simulink model "Channelizer_demo"  (R2023b)
settings: Solver=VariableStepAuto  StartTime=0.0  StopTime=inf  RelTol=1e-3
PostLoadFcn:
  | TT = numerictype(1,16,15);
  | FF = fimath('RoundingMethod','Nearest','OverflowAction','Saturate');
  | mdl = channelizer_init(TT, FF);
  | channelizer = channelizer_model(mdl, TT, FF );
  | Ts = 16*(7/4)/8.75e9;
  | ch_filt_coef = rcosdesign(0.22,4,28,'normal');
  | ch_filt_coef = 28 * ch_filt_coef / sum(ch_filt_coef(:));
  | channelizer_demo_init;
values from neighbouring files (symbols this model uses):
  ch0_en = 0    [channelizer_demo_init.m]    (also in init.m)
  ch0_qam = 0    [channelizer_demo_init.m]    (also in init.m)
  ch0_swp = 0    [channelizer_demo_init.m]    (also in init.m)
  ch10_en = 0    [channelizer_demo_init.m]    (also in init.m)
  ch10_qam = 0    [channelizer_demo_init.m]    (also in init.m)
  ch10_swp = 0    [channelizer_demo_init.m]    (also in init.m)
  ch11_en = 0    [channelizer_demo_init.m]    (also in init.m)
  ch11_qam = 0    [channelizer_demo_init.m]    (also in init.m)
  ch11_swp = 0    [channelizer_demo_init.m]    (also in init.m)
  ch12_en = 0    [channelizer_demo_init.m]    (also in init.m)
  ch12_qam = 0    [channelizer_demo_init.m]    (also in init.m)
  ch12_swp = 0    [channelizer_demo_init.m]    (also in init.m)
  ch13_en = 0    [channelizer_demo_init.m]    (also in init.m)
  ch13_qam = 0    [channelizer_demo_init.m]    (also in init.m)
  ch13_swp = 0    [channelizer_demo_init.m]    (also in init.m)
  ch14_en = 0    [channelizer_demo_init.m]    (also in init.m)
  ch14_qam = 0    [channelizer_demo_init.m]    (also in init.m)
  ch14_swp = 0    [channelizer_demo_init.m]    (also in init.m)
  ch15_en = 0    [channelizer_demo_init.m]    (also in init.m)
  ch15_qam = 0    [channelizer_demo_init.m]    (also in init.m)
  ch15_swp = 0    [channelizer_demo_init.m]    (also in init.m)
  ch1_en = 1    [channelizer_demo_init.m]    (also in init.m)
  ch1_qam = 0    [channelizer_demo_init.m]    (also in init.m)
  ch1_swp = 0    [channelizer_demo_init.m]    (also in init.m)
  ch2_en = 1    [channelizer_demo_init.m]    (also in init.m)
  ch2_qam = 0    [channelizer_demo_init.m]    (also in init.m)
  ch2_swp = 0    [channelizer_demo_init.m]    (also in init.m)
  ch3_en = 0    [channelizer_demo_init.m]    (also in init.m)
  ch3_qam = 0    [channelizer_demo_init.m]    (also in init.m)
  ch3_swp = 0    [channelizer_demo_init.m]    (also in init.m)
  ch4_en = 0    [channelizer_demo_init.m]    (also in init.m)
  ch4_qam = 0    [channelizer_demo_init.m]    (also in init.m)
  ch4_swp = 0    [channelizer_demo_init.m]    (also in init.m)
  ch5_en = 1    [channelizer_demo_init.m]    (also in init.m)
  ch5_qam = 1    [channelizer_demo_init.m]    (also in init.m)
  ch5_swp = 0    [channelizer_demo_init.m]    (also in init.m)
  ch6_en = 1    [channelizer_demo_init.m]    (also in init.m)
  ch6_qam = 1    [channelizer_demo_init.m]    (also in init.m)
  ch6_swp = 0    [channelizer_demo_init.m]    (also in init.m)
  ch7_en = 0    [channelizer_demo_init.m]    (also in init.m)
  ch7_qam = 0    [channelizer_demo_init.m]    (also in init.m)
  ch7_swp = 0    [channelizer_demo_init.m]    (also in init.m)
  ch8_en = 0    [channelizer_demo_init.m]    (also in init.m)
  ch8_qam = 0    [channelizer_demo_init.m]    (also in init.m)
  ch8_swp = 0    [channelizer_demo_init.m]    (also in init.m)
  ch9_en = 0    [channelizer_demo_init.m]    (also in init.m)
  ch9_qam = 0    [channelizer_demo_init.m]    (also in init.m)
  ch9_swp = 0    [channelizer_demo_init.m]    (also in init.m)
  spec1_ch = 1    [channelizer_demo_init.m]    (also in init.m)
  spec2_ch = 2    [channelizer_demo_init.m]    (also in init.m)
  spec3_ch = 5    [channelizer_demo_init.m]    (also in init.m)
  spec4_ch = 6    [channelizer_demo_init.m]    (also in init.m)
  swp_rate0 = 0    [channelizer_demo_init.m]    (also in init.m)
  swp_rate1 = 0    [channelizer_demo_init.m]    (also in init.m)
  swp_rate10 = 0    [channelizer_demo_init.m]    (also in init.m)
  swp_rate11 = 0    [channelizer_demo_init.m]    (also in init.m)
  swp_rate12 = 0    [channelizer_demo_init.m]    (also in init.m)
  swp_rate13 = 0    [channelizer_demo_init.m]    (also in init.m)
  swp_rate14 = 0    [channelizer_demo_init.m]    (also in init.m)
  swp_rate15 = 0    [channelizer_demo_init.m]    (also in init.m)
  swp_rate2 = 0    [channelizer_demo_init.m]    (also in init.m)
  swp_rate3 = 0    [channelizer_demo_init.m]    (also in init.m)
  swp_rate4 = 0    [channelizer_demo_init.m]    (also in init.m)
  swp_rate5 = 0    [channelizer_demo_init.m]    (also in init.m)
  swp_rate6 = 0    [channelizer_demo_init.m]    (also in init.m)
  swp_rate7 = 0    [channelizer_demo_init.m]    (also in init.m)
  swp_rate8 = 0    [channelizer_demo_init.m]    (also in init.m)
  swp_rate9 = 0    [channelizer_demo_init.m]    (also in init.m)
undefined symbols (not defined in the file or in its folder): S, vsva2197, xcvc1902
libraries: aieUtilities x39, aieBasic x34, dspswit3 x16, dspsigops x16, hlsBasic x3, vmcUtilities x1, commchan3 x1
(part 1 of 3)
settings Model: Creator=robg  LastModifiedBy=rbuz
settings DataIOCC: SaveFormat=Array  SaveOutput=off  SignalLogging=off  DSMLogging=off  SaveTime=off
settings OptimizationCC: ReuseModelBlockBuffer=off
settings DebuggingCC: ParameterOverflowMsg=none  ParameterPrecisionLossMsg=none  UnconnectedInputMsg=warning  UnconnectedOutputMsg=warning  UnconnectedLineMsg=warning
settings ModelReferenceCC: EnableRefExpFcnMdlSchedulingChecks=on
settings RTWCC: DLArmComputeVersion=19.05

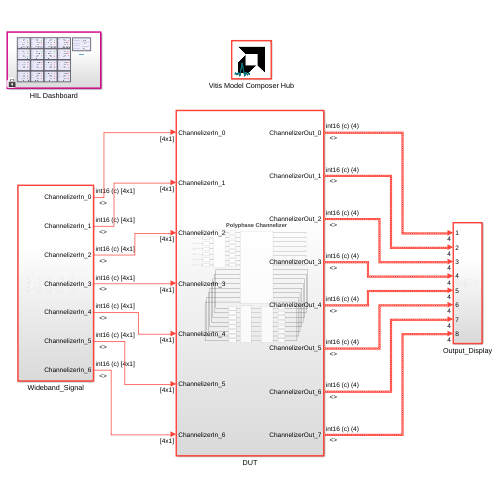
[thumbnail: Simulink's stored preview of the top-level diagram]
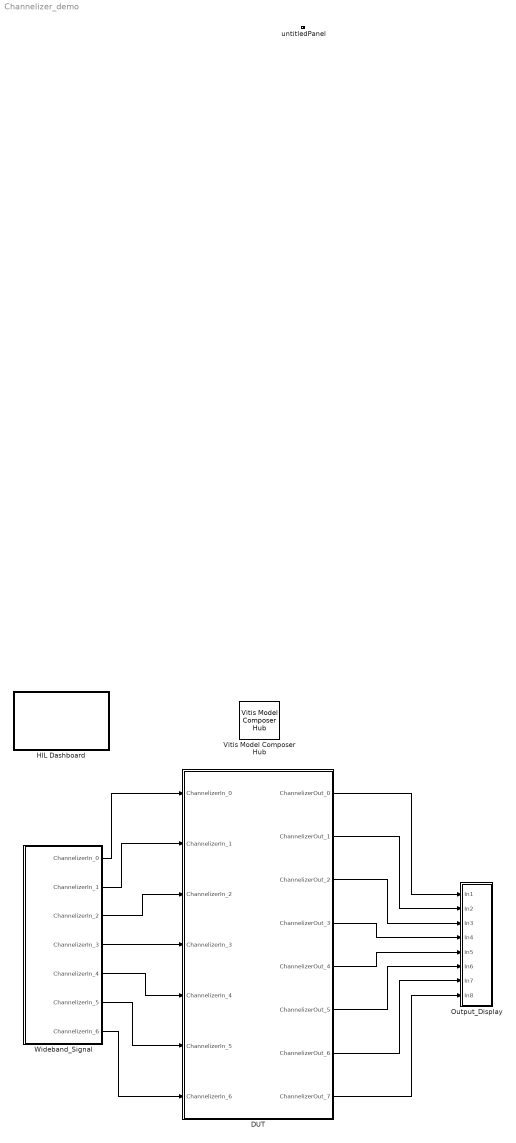
== system Channelizer_demo ==
  DUT : Subsystem
  HIL Dashboard : Subsystem
  Output_Display : Subsystem
  Vitis Model Composer Hub : vmcUtilities/Vitis Model Composer Hub  Tag=genX  CodeGeneration=off  SubsystemName=Channelizer  TargetDirectory=./code  exportDesign=off  analyzeDesign=off  validateDesignOnHw=off  ExportType=HW Code  IpVendor=xilinx.com  IpLibrary=hls  IpVersion=1.0  IpHWLanguage=Verilog  AieCompilerOptions={}  AieSimulatorOptions={}  CreateTestbench=off  TestbenchStackSize=10  RunRtlSim=off  RunCSim=off  RunAieSim=off  AieSimTimeout=50000  RunAieSimProfiling=off  LaunchVitisAnalyzer=off  PlotOutput=off  RunX86Sim=off  X86SimTimeout=10  GenHwImage=off  GenLibadfXo=off  GenHwValidationCode=off  PlatformType=Specify Platform  Platform=/proj/xbuilds/SWIP/2023.2_0918_2207/installs/lin64/Vitis/2023.2/base_platforms/xilinx_vck190_base_202320_1/xilinx_vck190_base_202320_1.xpfm  HwSystemType=Baremetal  HwValidationTarget=hw_emu  ProjDevice=Versal VCK190 Evaluation Platform (xcvc1902-vsva2197-2MP-e-S)  ProjDevicePart=xcvc1902-vsva2197-2MP-e-S  AIEType=AIE  SamplePeriod=-1  ClockFrequency=200  DataPathParallelism=1  xilinxfamily=versalaicore  part=xcvc1902  speed=-2MP-e-S  package=vsva2197  directory=./netlist  testbench=off  incr_netlist=off  synthesis_tool=Vivado  clock_wrapper=Clock Enables  dbl_ovrd=According to Block Masks  dcm_input_clock_period=10  sysclk_period=10  simulink_period=1  eval_field=0  LogFileName=/proj/xcoswmktg/robg/git/vmc_examples/gitent/Examples/AIENGINE_plus_PL/AIE_HLS/Channelizer/code/model_composer.log  NThreads=4
  Wideband_Signal : Subsystem
  untitledPanel : Subsystem  Tag=HiddenForWebPanel  IsWebBlockPanel=on
  wires:
  Wideband_Signal/7(ChannelizerIn_6) -> DUT/7(ChannelizerIn_6)
  Wideband_Signal/6(ChannelizerIn_5) -> DUT/6(ChannelizerIn_5)
  Wideband_Signal/5(ChannelizerIn_4) -> DUT/5(ChannelizerIn_4)
  Wideband_Signal/4(ChannelizerIn_3) -> DUT/4(ChannelizerIn_3)
  Wideband_Signal/3(ChannelizerIn_2) -> DUT/3(ChannelizerIn_2)
  Wideband_Signal/2(ChannelizerIn_1) -> DUT/2(ChannelizerIn_1)
  Wideband_Signal/1(ChannelizerIn_0) -> DUT/1(ChannelizerIn_0)
  DUT/1(ChannelizerOut_0) -> Output_Display/1(In1)
  DUT/2(ChannelizerOut_1) -> Output_Display/2(In2)
  DUT/3(ChannelizerOut_2) -> Output_Display/3(In3)
  DUT/4(ChannelizerOut_3) -> Output_Display/4(In4)
  DUT/5(ChannelizerOut_4) -> Output_Display/5(In5)
  DUT/6(ChannelizerOut_5) -> Output_Display/6(In6)
  DUT/7(ChannelizerOut_6) -> Output_Display/7(In7)
  DUT/8(ChannelizerOut_7) -> Output_Display/8(In8)

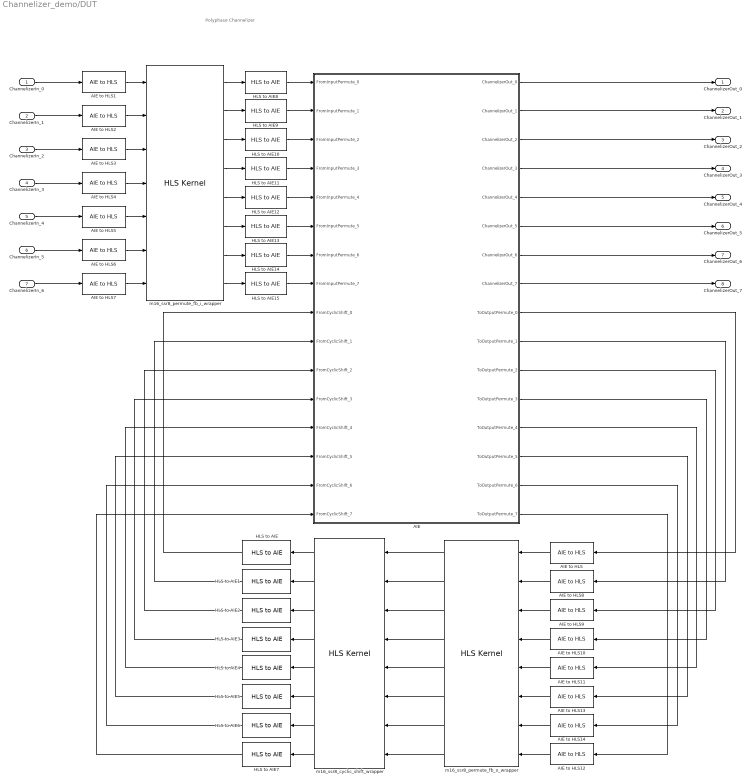
== system Channelizer_demo/DUT ==
  note: Polyphase Channelizer
  ChannelizerIn_0 : Inport
  ChannelizerIn_1 : Inport  Port=2
  ChannelizerIn_2 : Inport  Port=3
  ChannelizerIn_3 : Inport  Port=4
  ChannelizerIn_4 : Inport  Port=5
  ChannelizerIn_5 : Inport  Port=6
  ChannelizerIn_6 : Inport  Port=7
  AIE : Subsystem
  AIE to HLS{,1..14} (15 alike) : aieUtilities/AIE to HLS  OutputType=ufix128  OutputSize=1
  HLS to AIE{,1..15} (16 alike) : aieUtilities/HLS to AIE  OutputType=cint16  OutputSize=4
  m16_ssr8_cyclic_shift_wrapper : hlsBasic/HLS Kernel  PortNames={'return'; 'sig0_i'; 'sig1_i'; 'sig2_i'; 'sig3_i'; 'sig4_i'; 'sig5_i'; 'sig6_i'; 'sig7_i'; 'sig0_o'; 'sig1_o'; 'sig2_o'; 'sig3_o'; 'sig4_o'; 'sig5_o'; 'sig6_o'; 'sig7_o'}  PortSerializedTypes={'{Bv}'; '{R{Thls::stream{2{t{Tap_uint{1{t{}128}}}}{t{}0}}}}'; '{R{Thls::stream{2{t{Tap_uint{1{t{}128}}}}{t{}0}}}}'; '{R{Thls::stream{2{t{Tap_uint{1{t{}128}}}}{t{}0}}}}'; '{R{Thls::stream{2{t{Tap_uint{1{t{}128}}}}{t{}0}}}}'; '{R{Thls::stream{2{t{Tap_uint{1{t{}128}}}}{t{}0}}}}'; '{R{Thls::stream{2{t{Tap_uint{1{t{}128}}}}{t{}0}}}}'; '{R{Thls::stream{2{t{Tap_uint{1{t{}128}}}}{t{}0}}}}'; '{R{Thls::stream{2{t{Tap_uint{1{t{}128}}}}{t{}0}}}}'; '{R{Thls::stream{2{t{Tap_uint{1{t{}128}}}}{t{}0}}}}'; '{R{Thls::stream{2{t{Tap_uint{1{t{}128}}}}{t{}0}}}}'; '{R{Thls::stream{2{t{Tap_uint{1{t{}128}}}}{t{}0}}}}'; '{R{Thls::stream{2{t{Tap_uint{1{t{}128}}}}{t{}0}}}}'; '{R{Thls::stream{2{t{Tap_uint{1{t{}128}}}}{t{}0}}}}'; '{R{Thls::stream{2{t{Tap_uint{1{t{}128}}}}{t{}0}}}}'; '{R{Thls::stream{2{t{Tap_uint{1{t{}128}}}}{t{}0}}}}'; '{R{Thls::stream{2{t{Tap_uint{1{t{}128}}}}{t{}0}}}}'}  FunctionTemplateSpecKind=none  FunctionTemplateParamNames={}  FunctionTemplateParamKinds={}  FunctionTemplateParamTypes={}  FunctionTemplateParamValues={}  PortSynchronicities={'auto'; 'auto'; 'auto'; 'auto'; 'auto'; 'auto'; 'auto'; 'auto'; 'auto'; 'auto'; 'auto'; 'auto'; 'auto'; 'auto'; 'auto'; 'auto'}  PortSignalSizes={0.000000000000000000e+00; 0.000000000000000000e+00; 0.000000000000000000e+00; 0.000000000000000000e+00; 0.000000000000000000e+00; 0.000000000000000000e+00; 0.000000000000000000e+00; 0.000000000000000000e+00; 1.000000000000000000e+00; 1.000000000000000000e+00; 1.000000000000000000e+00; 1.000000000000000000e+00; 1.000000000000000000e+00; 1.000000000000000000e+00; 1.000000000000000000e+00; 1.000000000000000000e+00}  PortParameterValues={}  FunctionTemplateParams={}  FunctionTemplateParamsEnables={}  FunctionTemplateParamsVisible=off  FunctionDeclTypeOptions=C[1 1]@t7@<empty>  PortAttributesTable={ 'Input', 'sig0_i', 'hls::stream< ap_uint< 128 >, 0 > &', '', ''; 'Input', 'sig1_i', 'hls::stream< ap_uint< 128 >, 0 > &', '', ''; 'Input', 'sig2_i', 'hls::stream< ap_uint< 128 >, 0 > &', '', ''; 'Input', 'sig3_i', 'hls::stream< ap_uint< 128 >, 0 > &', '', ''; 'Input', 'sig4_i', 'hls::stream< ap_uint< 128 >, 0 > &', '', ''; 'Input', 'sig5_i', 'hls::stream< ap_uint< 128 >, 0 > &', '', ''; 'Input', 'sig6_i', 'hls::stream< ap_uint< 128 >, 0 > &', '', ''; 'Input', 'sig7_i', 'hls::stream< ap_uint< 128 >, 0 > &', '', ''; 'Output', 'sig0_o', 'hls::stream< ap_uint< 128 >, 0 > &', '', '1'; 'Output', 'sig1_o', 'hls::stream< ap_uint< 128 >, 0 > &', '', '1'; 'Output', 'sig2_o', 'hls::stream< ap_uint< 128 >, 0 > &', '', '1'; 'Output', 'sig3_o', 'hls::stream< ap_uint< 128 >, 0 > &', '', '1'; 'Output', 'sig4_o', 'hls::stream< ap_uint< 128 >, 0 > &', '', '1'; 'Output', 'sig5_o', 'hls::stream< ap_uint< 128 >, 0 > &', '', '1'; 'Output', 'sig6_o', 'hls::stream< ap_uint< 128 >, 0 > &', '', '1'; 'Output', 'sig7_o', 'hls::stream< ap_uint< 128 >, 0 > &', '', '1' }  PortAttributesEnablement={'off', 'off', 'off', 'off', 'off';'off', 'off', 'off', 'off', 'off';'off', 'off', 'off', 'off', 'off';'off', 'off', 'off', 'off', 'off';'off', 'off', 'off', 'off', 'off';'off', 'off', 'off', 'off', 'off';'off', 'off', 'off', 'off', 'off';'off', 'off', 'off', 'off', 'off';'off', 'off', 'off', 'off', 'on';'off', 'off', 'off', 'off', 'on';'off', 'off', 'off', 'off', 'on';'off', 'off', 'off', 'off', 'on';'off', 'off', 'off', 'off', 'on';'off', 'off', 'off', 'off', 'on';'off', 'off', 'off', 'off', 'on';'off', 'off', 'off', 'off', 'on'}  PortParametersTable={}  SampleTime=-1  PortDirectionTable={ 'sig0_i', 'hls::stream< ap_uint< 128 >, 0 > &', 'Input', 'Port'; 'sig1_i', 'hls::stream< ap_uint< 128 >, 0 > &', 'Input', 'Port'; 'sig2_i', 'hls::stream< ap_uint< 128 >, 0 > &', 'Input', 'Port'; 'sig3_i', 'hls::stream< ap_uint< 128 >, 0 > &', 'Input', 'Port'; 'sig4_i', 'hls::stream< ap_uint< 128 >, 0 > &', 'Input', 'Port'; 'sig5_i', 'hls::stream< ap_uint< 128 >, 0 > &', 'Input', 'Port'; 'sig6_i', 'hls::stream< ap_uint< 128 >, 0 > &', 'Input', 'Port'; 'sig7_i', 'hls::stream< ap_uint< 128 >, 0 > &', 'Input', 'Port'; 'sig0_o', 'hls::stream< ap_uint< 128 >, 0 > &', 'Output', 'Port'; 'sig1_o', 'hls::stream< ap_uint< 128 >, 0 > &', 'Output', 'Port'; 'sig2_o', 'hls::stream< ap_uint< 128 >, 0 > &', 'Output', 'Port'; 'sig3_o', 'hls::stream< ap_uint< 128 >, 0 > &', 'Output', 'Port'; 'sig4_o', 'hls::stream< ap_uint< 128 >, 0 > &', 'Output', 'Port'; 'sig5_o', 'hls::stream< ap_uint< 128 >, 0 > &', 'Output', 'Port'; 'sig6_o', 'hls::stream< ap_uint< 128 >, 0 > &', 'Output', 'Port'; 'sig7_o', 'hls::stream< ap_uint< 128 >, 0 > &', 'Output', 'Port' }  PortDirectionTabVisible=on  ArgDirections={1.000000000000000000e+00; 1.000000000000000000e+00; 1.000000000000000000e+00; 1.000000000000000000e+00; 1.000000000000000000e+00; 1.000000000000000000e+00; 1.000000000000000000e+00; 1.000000000000000000e+00; 2.000000000000000000e+00; 2.000000000000000000e+00; 2.000000000000000000e+00; 2.000000000000000000e+00; 2.000000000000000000e+00; 2.000000000000000000e+00; 2.000000000000000000e+00; 2.000000000000000000e+00}  ArgInterfaceTypes={1.000000000000000000e+00; 1.000000000000000000e+00; 1.000000000000000000e+00; 1.000000000000000000e+00; 1.000000000000000000e+00; 1.000000000000000000e+00; 1.000000000000000000e+00; 1.000000000000000000e+00; 1.000000000000000000e+00; 1.000000000000000000e+00; 1.000000000000000000e+00; 1.000000000000000000e+00; 1.000000000000000000e+00; 1.000000000000000000e+00; 1.000000000000000000e+00; 1.000000000000000000e+00}  FunctionIndex=1  FormalArgDecls={'hls::stream< ap_uint< 128 >, 0 > & sig0_i', 'hls::stream< ap_uint< 128 >, 0 > & sig1_i', 'hls::stream< ap_uint< 128 >, 0 > & sig2_i', 'hls::stream< ap_uint< 128 >, 0 > & sig3_i', 'hls::stream< ap_uint< 128 >, 0 > & sig4_i', 'hls::stream< ap_uint< 128 >, 0 > & sig5_i', 'hls::stream< ap_uint< 128 >, 0 > & sig6_i', 'hls::stream< ap_uint< 128 >, 0 > & sig7_i', 'hls::stream< ap_uint< 128 >, 0 > & sig0_o', 'hls::stream< ap_uint< 128 >, 0 > & sig1_o', 'hls::stream< ap_uint< 128 >, 0 > & sig2_o', 'hls::stream< ap_uint< 128 >, 0 > & sig3_o', 'hls::stream< ap_uint< 128 >, 0 > & sig4_o', 'hls::stream< ap_uint< 128 >, 0 > & sig5_o', 'hls::stream< ap_uint< 128 >, 0 > & sig6_o', 'hls::stream< ap_uint< 128 >, 0 > & sig7_o'}  SimLibPath=''  FunctionTabVisible=on  FunctionDescription=void m16_ssr8_cyclic_shift_wrapper(hls::stream< ap_uint< 128 >, 0 > & sig0_i, hls::stream< ap_uint< 128 >, 0 > & sig1_i, hls::stream< ap_uint< 128 >, 0 > & sig2_i, hls::stream< ap_uint< 128 >, 0 > & sig3_i, hls::stream< ap_uint< 128 >, 0 > & sig4_i, hls::stream< ap_uint< 128 >, 0 > & sig5_i, hls::stream< ap_uint< 128 >, 0 > & sig6_i, hls::stream< ap_uint< 128 >, 0 > & sig7_i, hls::stream< ap_uint< 128 >, 0 > & sig0_o, hls::stream< ap_uint< 128 >, 0 > & sig1_o, hls::stream< ap_uint< 128 >, 0 > & sig2_o, hls::stream< ap_uint< 128 >, 0 > & sig3_o, hls::stream< ap_uint< 128 >, 0 > & sig4_o, hls::stream< ap_uint< 128 >, 0 > & sig5_o, hls::stream< ap_uint< 128 >, 0 > & sig6_o, hls::stream< ap_uint< 128 >, 0 > & sig7_o)  blockJsonConstraints=[]  deprecateConstraints=0  KernelHeaderFile=hls/m16_ssr8_cyclic_shift.h  KernelFunction=m16_ssr8_cyclic_shift_wrapper  KernelFunctionSelect=<empty>  KernelSourceFile=hls/m16_ssr8_cyclic_shift.cpp  KernelSearchPaths={}  PreProcOptions={}
  m16_ssr8_permute_fb_i_wrapper : hlsBasic/HLS Kernel  PortNames={'return'; 'sig0_i'; 'sig1_i'; 'sig2_i'; 'sig3_i'; 'sig4_i'; 'sig5_i'; 'sig6_i'; 'sig0_o'; 'sig1_o'; 'sig2_o'; 'sig3_o'; 'sig4_o'; 'sig5_o'; 'sig6_o'; 'sig7_o'}  PortSerializedTypes={'{Bv}'; '{R{Thls::stream{2{t{Tap_uint{1{t{}128}}}}{t{}0}}}}'; '{R{Thls::stream{2{t{Tap_uint{1{t{}128}}}}{t{}0}}}}'; '{R{Thls::stream{2{t{Tap_uint{1{t{}128}}}}{t{}0}}}}'; '{R{Thls::stream{2{t{Tap_uint{1{t{}128}}}}{t{}0}}}}'; '{R{Thls::stream{2{t{Tap_uint{1{t{}128}}}}{t{}0}}}}'; '{R{Thls::stream{2{t{Tap_uint{1{t{}128}}}}{t{}0}}}}'; '{R{Thls::stream{2{t{Tap_uint{1{t{}128}}}}{t{}0}}}}'; '{R{Thls::stream{2{t{Tap_uint{1{t{}128}}}}{t{}0}}}}'; '{R{Thls::stream{2{t{Tap_uint{1{t{}128}}}}{t{}0}}}}'; '{R{Thls::stream{2{t{Tap_uint{1{t{}128}}}}{t{}0}}}}'; '{R{Thls::stream{2{t{Tap_uint{1{t{}128}}}}{t{}0}}}}'; '{R{Thls::stream{2{t{Tap_uint{1{t{}128}}}}{t{}0}}}}'; '{R{Thls::stream{2{t{Tap_uint{1{t{}128}}}}{t{}0}}}}'; '{R{Thls::stream{2{t{Tap_uint{1{t{}128}}}}{t{}0}}}}'; '{R{Thls::stream{2{t{Tap_uint{1{t{}128}}}}{t{}0}}}}'}  FunctionTemplateSpecKind=none  FunctionTemplateParamNames={}  FunctionTemplateParamKinds={}  FunctionTemplateParamTypes={}  FunctionTemplateParamValues={}  PortSynchronicities={'auto'; 'auto'; 'auto'; 'auto'; 'auto'; 'auto'; 'auto'; 'auto'; 'auto'; 'auto'; 'auto'; 'auto'; 'auto'; 'auto'; 'auto'}  PortSignalSizes={0.000000000000000000e+00; 0.000000000000000000e+00; 0.000000000000000000e+00; 0.000000000000000000e+00; 0.000000000000000000e+00; 0.000000000000000000e+00; 0.000000000000000000e+00; 1.000000000000000000e+00; 1.000000000000000000e+00; 1.000000000000000000e+00; 1.000000000000000000e+00; 1.000000000000000000e+00; 1.000000000000000000e+00; 1.000000000000000000e+00; 1.000000000000000000e+00}  PortParameterValues={}  FunctionTemplateParams={}  FunctionTemplateParamsEnables={}  FunctionTemplateParamsVisible=off  FunctionDeclTypeOptions=C[1 1]@t7@<empty>  PortAttributesTable={ 'Input', 'sig0_i', 'hls::stream< ap_uint< 128 >, 0 > &', '', ''; 'Input', 'sig1_i', 'hls::stream< ap_uint< 128 >, 0 > &', '', ''; 'Input', 'sig2_i', 'hls::stream< ap_uint< 128 >, 0 > &', '', ''; 'Input', 'sig3_i', 'hls::stream< ap_uint< 128 >, 0 > &', '', ''; 'Input', 'sig4_i', 'hls::stream< ap_uint< 128 >, 0 > &', '', ''; 'Input', 'sig5_i', 'hls::stream< ap_uint< 128 >, 0 > &', '', ''; 'Input', 'sig6_i', 'hls::stream< ap_uint< 128 >, 0 > &', '', ''; 'Output', 'sig0_o', 'hls::stream< ap_uint< 128 >, 0 > &', '', '1'; 'Output', 'sig1_o', 'hls::stream< ap_uint< 128 >, 0 > &', '', '1'; 'Output', 'sig2_o', 'hls::stream< ap_uint< 128 >, 0 > &', '', '1'; 'Output', 'sig3_o', 'hls::stream< ap_uint< 128 >, 0 > &', '', '1'; 'Output', 'sig4_o', 'hls::stream< ap_uint< 128 >, 0 > &', '', '1'; 'Output', 'sig5_o', 'hls::stream< ap_uint< 128 >, 0 > &', '', '1'; 'Output', 'sig6_o', 'hls::stream< ap_uint< 128 >, 0 > &', '', '1'; 'Output', 'sig7_o', 'hls::stream< ap_uint< 128 >, 0 > &', '', '1' }  PortAttributesEnablement={'off', 'off', 'off', 'off', 'off';'off', 'off', 'off', 'off', 'off';'off', 'off', 'off', 'off', 'off';'off', 'off', 'off', 'off', 'off';'off', 'off', 'off', 'off', 'off';'off', 'off', 'off', 'off', 'off';'off', 'off', 'off', 'off', 'off';'off', 'off', 'off', 'off', 'on';'off', 'off', 'off', 'off', 'on';'off', 'off', 'off', 'off', 'on';'off', 'off', 'off', 'off', 'on';'off', 'off', 'off', 'off', 'on';'off', 'off', 'off', 'off', 'on';'off', 'off', 'off', 'off', 'on';'off', 'off', 'off', 'off', 'on'}  PortParametersTable={}  SampleTime=-1  PortDirectionTable={ 'sig0_i', 'hls::stream< ap_uint< 128 >, 0 > &', 'Input', 'Port'; 'sig1_i', 'hls::stream< ap_uint< 128 >, 0 > &', 'Input', 'Port'; 'sig2_i', 'hls::stream< ap_uint< 128 >, 0 > &', 'Input', 'Port'; 'sig3_i', 'hls::stream< ap_uint< 128 >, 0 > &', 'Input', 'Port'; 'sig4_i', 'hls::stream< ap_uint< 128 >, 0 > &', 'Input', 'Port'; 'sig5_i', 'hls::stream< ap_uint< 128 >, 0 > &', 'Input', 'Port'; 'sig6_i', 'hls::stream< ap_uint< 128 >, 0 > &', 'Input', 'Port'; 'sig0_o', 'hls::stream< ap_uint< 128 >, 0 > &', 'Output', 'Port'; 'sig1_o', 'hls::stream< ap_uint< 128 >, 0 > &', 'Output', 'Port'; 'sig2_o', 'hls::stream< ap_uint< 128 >, 0 > &', 'Output', 'Port'; 'sig3_o', 'hls::stream< ap_uint< 128 >, 0 > &', 'Output', 'Port'; 'sig4_o', 'hls::stream< ap_uint< 128 >, 0 > &', 'Output', 'Port'; 'sig5_o', 'hls::stream< ap_uint< 128 >, 0 > &', 'Output', 'Port'; 'sig6_o', 'hls::stream< ap_uint< 128 >, 0 > &', 'Output', 'Port'; 'sig7_o', 'hls::stream< ap_uint< 128 >, 0 > &', 'Output', 'Port' }  PortDirectionTabVisible=on  ArgDirections={1.000000000000000000e+00; 1.000000000000000000e+00; 1.000000000000000000e+00; 1.000000000000000000e+00; 1.000000000000000000e+00; 1.000000000000000000e+00; 1.000000000000000000e+00; 2.000000000000000000e+00; 2.000000000000000000e+00; 2.000000000000000000e+00; 2.000000000000000000e+00; 2.000000000000000000e+00; 2.000000000000000000e+00; 2.000000000000000000e+00; 2.000000000000000000e+00}  ArgInterfaceTypes={1.000000000000000000e+00; 1.000000000000000000e+00; 1.000000000000000000e+00; 1.000000000000000000e+00; 1.000000000000000000e+00; 1.000000000000000000e+00; 1.000000000000000000e+00; 1.000000000000000000e+00; 1.000000000000000000e+00; 1.000000000000000000e+00; 1.000000000000000000e+00; 1.000000000000000000e+00; 1.000000000000000000e+00; 1.000000000000000000e+00; 1.000000000000000000e+00}  FunctionIndex=1  FormalArgDecls={'hls::stream< ap_uint< 128 >, 0 > & sig0_i', 'hls::stream< ap_uint< 128 >, 0 > & sig1_i', 'hls::stream< ap_uint< 128 >, 0 > & sig2_i', 'hls::stream< ap_uint< 128 >, 0 > & sig3_i', 'hls::stream< ap_uint< 128 >, 0 > & sig4_i', 'hls::stream< ap_uint< 128 >, 0 > & sig5_i', 'hls::stream< ap_uint< 128 >, 0 > & sig6_i', 'hls::stream< ap_uint< 128 >, 0 > & sig0_o', 'hls::stream< ap_uint< 128 >, 0 > & sig1_o', 'hls::stream< ap_uint< 128 >, 0 > & sig2_o', 'hls::stream< ap_uint< 128 >, 0 > & sig3_o', 'hls::stream< ap_uint< 128 >, 0 > & sig4_o', 'hls::stream< ap_uint< 128 >, 0 > & sig5_o', 'hls::stream< ap_uint< 128 >, 0 > & sig6_o', 'hls::stream< ap_uint< 128 >, 0 > & sig7_o'}  SimLibPath=''  FunctionTabVisible=on  FunctionDescription=void m16_ssr8_permute_fb_i_wrapper(hls::stream< ap_uint< 128 >, 0 > & sig0_i, hls::stream< ap_uint< 128 >, 0 > & sig1_i, hls::stream< ap_uint< 128 >, 0 > & sig2_i, hls::stream< ap_uint< 128 >, 0 > & sig3_i, hls::stream< ap_uint< 128 >, 0 > & sig4_i, hls::stream< ap_uint< 128 >, 0 > & sig5_i, hls::stream< ap_uint< 128 >, 0 > & sig6_i, hls::stream< ap_uint< 128 >, 0 > & sig0_o, hls::stream< ap_uint< 128 >, 0 > & sig1_o, hls::stream< ap_uint< 128 >, 0 > & sig2_o, hls::stream< ap_uint< 128 >, 0 > & sig3_o, hls::stream< ap_uint< 128 >, 0 > & sig4_o, hls::stream< ap_uint< 128 >, 0 > & sig5_o, hls::stream< ap_uint< 128 >, 0 > & sig6_o, hls::stream< ap_uint< 128 >, 0 > & sig7_o)  blockJsonConstraints=[]  deprecateConstraints=0  KernelHeaderFile=hls/m16_ssr8_permute_fb_i.h  KernelFunction=m16_ssr8_permute_fb_i_wrapper  KernelFunctionSelect=<empty>  KernelSourceFile=hls/m16_ssr8_permute_fb_i.cpp  KernelSearchPaths={}  PreProcOptions={}
  m16_ssr8_permute_fb_o_wrapper : hlsBasic/HLS Kernel  PortNames={'return'; 'sig0_i'; 'sig1_i'; 'sig2_i'; 'sig3_i'; 'sig4_i'; 'sig5_i'; 'sig6_i'; 'sig7_i'; 'sig0_o'; 'sig1_o'; 'sig2_o'; 'sig3_o'; 'sig4_o'; 'sig5_o'; 'sig6_o'; 'sig7_o'}  PortSerializedTypes={'{Bv}'; '{R{Thls::stream{2{t{Tap_uint{1{t{}128}}}}{t{}0}}}}'; '{R{Thls::stream{2{t{Tap_uint{1{t{}128}}}}{t{}0}}}}'; '{R{Thls::stream{2{t{Tap_uint{1{t{}128}}}}{t{}0}}}}'; '{R{Thls::stream{2{t{Tap_uint{1{t{}128}}}}{t{}0}}}}'; '{R{Thls::stream{2{t{Tap_uint{1{t{}128}}}}{t{}0}}}}'; '{R{Thls::stream{2{t{Tap_uint{1{t{}128}}}}{t{}0}}}}'; '{R{Thls::stream{2{t{Tap_uint{1{t{}128}}}}{t{}0}}}}'; '{R{Thls::stream{2{t{Tap_uint{1{t{}128}}}}{t{}0}}}}'; '{R{Thls::stream{2{t{Tap_uint{1{t{}128}}}}{t{}0}}}}'; '{R{Thls::stream{2{t{Tap_uint{1{t{}128}}}}{t{}0}}}}'; '{R{Thls::stream{2{t{Tap_uint{1{t{}128}}}}{t{}0}}}}'; '{R{Thls::stream{2{t{Tap_uint{1{t{}128}}}}{t{}0}}}}'; '{R{Thls::stream{2{t{Tap_uint{1{t{}128}}}}{t{}0}}}}'; '{R{Thls::stream{2{t{Tap_uint{1{t{}128}}}}{t{}0}}}}'; '{R{Thls::stream{2{t{Tap_uint{1{t{}128}}}}{t{}0}}}}'; '{R{Thls::stream{2{t{Tap_uint{1{t{}128}}}}{t{}0}}}}'}  FunctionTemplateSpecKind=none  FunctionTemplateParamNames={}  FunctionTemplateParamKinds={}  FunctionTemplateParamTypes={}  FunctionTemplateParamValues={}  PortSynchronicities={'auto'; 'auto'; 'auto'; 'auto'; 'auto'; 'auto'; 'auto'; 'auto'; 'auto'; 'auto'; 'auto'; 'auto'; 'auto'; 'auto'; 'auto'; 'auto'}  PortSignalSizes={0.000000000000000000e+00; 0.000000000000000000e+00; 0.000000000000000000e+00; 0.000000000000000000e+00; 0.000000000000000000e+00; 0.000000000000000000e+00; 0.000000000000000000e+00; 0.000000000000000000e+00; 1.000000000000000000e+00; 1.000000000000000000e+00; 1.000000000000000000e+00; 1.000000000000000000e+00; 1.000000000000000000e+00; 1.000000000000000000e+00; 1.000000000000000000e+00; 1.000000000000000000e+00}  PortParameterValues={}  FunctionTemplateParams={}  FunctionTemplateParamsEnables={}  FunctionTemplateParamsVisible=off  FunctionDeclTypeOptions=C[1 1]@t7@<empty>  PortAttributesTable={ 'Input', 'sig0_i', 'hls::stream< ap_uint< 128 >, 0 > &', '', ''; 'Input', 'sig1_i', 'hls::stream< ap_uint< 128 >, 0 > &', '', ''; 'Input', 'sig2_i', 'hls::stream< ap_uint< 128 >, 0 > &', '', ''; 'Input', 'sig3_i', 'hls::stream< ap_uint< 128 >, 0 > &', '', ''; 'Input', 'sig4_i', 'hls::stream< ap_uint< 128 >, 0 > &', '', ''; 'Input', 'sig5_i', 'hls::stream< ap_uint< 128 >, 0 > &', '', ''; 'Input', 'sig6_i', 'hls::stream< ap_uint< 128 >, 0 > &', '', ''; 'Input', 'sig7_i', 'hls::stream< ap_uint< 128 >, 0 > &', '', ''; 'Output', 'sig0_o', 'hls::stream< ap_uint< 128 >, 0 > &', '', '1'; 'Output', 'sig1_o', 'hls::stream< ap_uint< 128 >, 0 > &', '', '1'; 'Output', 'sig2_o', 'hls::stream< ap_uint< 128 >, 0 > &', '', '1'; 'Output', 'sig3_o', 'hls::stream< ap_uint< 128 >, 0 > &', '', '1'; 'Output', 'sig4_o', 'hls::stream< ap_uint< 128 >, 0 > &', '', '1'; 'Output', 'sig5_o', 'hls::stream< ap_uint< 128 >, 0 > &', '', '1'; 'Output', 'sig6_o', 'hls::stream< ap_uint< 128 >, 0 > &', '', '1'; 'Output', 'sig7_o', 'hls::stream< ap_uint< 128 >, 0 > &', '', '1' }  PortAttributesEnablement={'off', 'off', 'off', 'off', 'off';'off', 'off', 'off', 'off', 'off';'off', 'off', 'off', 'off', 'off';'off', 'off', 'off', 'off', 'off';'off', 'off', 'off', 'off', 'off';'off', 'off', 'off', 'off', 'off';'off', 'off', 'off', 'off', 'off';'off', 'off', 'off', 'off', 'off';'off', 'off', 'off', 'off', 'on';'off', 'off', 'off', 'off', 'on';'off', 'off', 'off', 'off', 'on';'off', 'off', 'off', 'off', 'on';'off', 'off', 'off', 'off', 'on';'off', 'off', 'off', 'off', 'on';'off', 'off', 'off', 'off', 'on';'off', 'off', 'off', 'off', 'on'}  PortParametersTable={}  SampleTime=-1  PortDirectionTable={ 'sig0_i', 'hls::stream< ap_uint< 128 >, 0 > &', 'Input', 'Port'; 'sig1_i', 'hls::stream< ap_uint< 128 >, 0 > &', 'Input', 'Port'; 'sig2_i', 'hls::stream< ap_uint< 128 >, 0 > &', 'Input', 'Port'; 'sig3_i', 'hls::stream< ap_uint< 128 >, 0 > &', 'Input', 'Port'; 'sig4_i', 'hls::stream< ap_uint< 128 >, 0 > &', 'Input', 'Port'; 'sig5_i', 'hls::stream< ap_uint< 128 >, 0 > &', 'Input', 'Port'; 'sig6_i', 'hls::stream< ap_uint< 128 >, 0 > &', 'Input', 'Port'; 'sig7_i', 'hls::stream< ap_uint< 128 >, 0 > &', 'Input', 'Port'; 'sig0_o', 'hls::stream< ap_uint< 128 >, 0 > &', 'Output', 'Port'; 'sig1_o', 'hls::stream< ap_uint< 128 >, 0 > &', 'Output', 'Port'; 'sig2_o', 'hls::stream< ap_uint< 128 >, 0 > &', 'Output', 'Port'; 'sig3_o', 'hls::stream< ap_uint< 128 >, 0 > &', 'Output', 'Port'; 'sig4_o', 'hls::stream< ap_uint< 128 >, 0 > &', 'Output', 'Port'; 'sig5_o', 'hls::stream< ap_uint< 128 >, 0 > &', 'Output', 'Port'; 'sig6_o', 'hls::stream< ap_uint< 128 >, 0 > &', 'Output', 'Port'; 'sig7_o', 'hls::stream< ap_uint< 128 >, 0 > &', 'Output', 'Port' }  PortDirectionTabVisible=on  ArgDirections={1.000000000000000000e+00; 1.000000000000000000e+00; 1.000000000000000000e+00; 1.000000000000000000e+00; 1.000000000000000000e+00; 1.000000000000000000e+00; 1.000000000000000000e+00; 1.000000000000000000e+00; 2.000000000000000000e+00; 2.000000000000000000e+00; 2.000000000000000000e+00; 2.000000000000000000e+00; 2.000000000000000000e+00; 2.000000000000000000e+00; 2.000000000000000000e+00; 2.000000000000000000e+00}  ArgInterfaceTypes={1.000000000000000000e+00; 1.000000000000000000e+00; 1.000000000000000000e+00; 1.000000000000000000e+00; 1.000000000000000000e+00; 1.000000000000000000e+00; 1.000000000000000000e+00; 1.000000000000000000e+00; 1.000000000000000000e+00; 1.000000000000000000e+00; 1.000000000000000000e+00; 1.000000000000000000e+00; 1.000000000000000000e+00; 1.000000000000000000e+00; 1.000000000000000000e+00; 1.000000000000000000e+00}  FunctionIndex=1  FormalArgDecls={'hls::stream< ap_uint< 128 >, 0 > & sig0_i', 'hls::stream< ap_uint< 128 >, 0 > & sig1_i', 'hls::stream< ap_uint< 128 >, 0 > & sig2_i', 'hls::stream< ap_uint< 128 >, 0 > & sig3_i', 'hls::stream< ap_uint< 128 >, 0 > & sig4_i', 'hls::stream< ap_uint< 128 >, 0 > & sig5_i', 'hls::stream< ap_uint< 128 >, 0 > & sig6_i', 'hls::stream< ap_uint< 128 >, 0 > & sig7_i', 'hls::stream< ap_uint< 128 >, 0 > & sig0_o', 'hls::stream< ap_uint< 128 >, 0 > & sig1_o', 'hls::stream< ap_uint< 128 >, 0 > & sig2_o', 'hls::stream< ap_uint< 128 >, 0 > & sig3_o', 'hls::stream< ap_uint< 128 >, 0 > & sig4_o', 'hls::stream< ap_uint< 128 >, 0 > & sig5_o', 'hls::stream< ap_uint< 128 >, 0 > & sig6_o', 'hls::stream< ap_uint< 128 >, 0 > & sig7_o'}  SimLibPath=''  FunctionTabVisible=on  FunctionDescription=void m16_ssr8_permute_fb_o_wrapper(hls::stream< ap_uint< 128 >, 0 > & sig0_i, hls::stream< ap_uint< 128 >, 0 > & sig1_i, hls::stream< ap_uint< 128 >, 0 > & sig2_i, hls::stream< ap_uint< 128 >, 0 > & sig3_i, hls::stream< ap_uint< 128 >, 0 > & sig4_i, hls::stream< ap_uint< 128 >, 0 > & sig5_i, hls::stream< ap_uint< 128 >, 0 > & sig6_i, hls::stream< ap_uint< 128 >, 0 > & sig7_i, hls::stream< ap_uint< 128 >, 0 > & sig0_o, hls::stream< ap_uint< 128 >, 0 > & sig1_o, hls::stream< ap_uint< 128 >, 0 > & sig2_o, hls::stream< ap_uint< 128 >, 0 > & sig3_o, hls::stream< ap_uint< 128 >, 0 > & sig4_o, hls::stream< ap_uint< 128 >, 0 > & sig5_o, hls::stream< ap_uint< 128 >, 0 > & sig6_o, hls::stream< ap_uint< 128 >, 0 > & sig7_o)  blockJsonConstraints=[]  deprecateConstraints=0  KernelHeaderFile=hls/m16_ssr8_permute_fb_o.h  KernelFunction=m16_ssr8_permute_fb_o_wrapper  KernelFunctionSelect=<empty>  KernelSourceFile=hls/m16_ssr8_permute_fb_o.cpp  KernelSearchPaths={}  PreProcOptions={}
  ChannelizerOut_0 : Outport
  ChannelizerOut_1 : Outport  Port=2
  ChannelizerOut_2 : Outport  Port=3
  ChannelizerOut_3 : Outport  Port=4
  ChannelizerOut_4 : Outport  Port=5
  ChannelizerOut_5 : Outport  Port=6
  ChannelizerOut_6 : Outport  Port=7
  ChannelizerOut_7 : Outport  Port=8
  wires:
  m16_ssr8_cyclic_shift_wrapper/1 -> HLS to AIE/1
  m16_ssr8_cyclic_shift_wrapper/8 -> HLS to AIE7/1
  m16_ssr8_cyclic_shift_wrapper/6 -> HLS to AIE5/1
  m16_ssr8_cyclic_shift_wrapper/4 -> HLS to AIE3/1
  m16_ssr8_cyclic_shift_wrapper/7 -> HLS to AIE6/1
  m16_ssr8_cyclic_shift_wrapper/3 -> HLS to AIE2/1
  m16_ssr8_cyclic_shift_wrapper/2 -> HLS to AIE1/1
  m16_ssr8_cyclic_shift_wrapper/5 -> HLS to AIE4/1
  AIE/9(ToOutputPermute_0) -> AIE to HLS/1
  AIE/10(ToOutputPermute_1) -> AIE to HLS8/1
  AIE/11(ToOutputPermute_2) -> AIE to HLS9/1
  AIE/12(ToOutputPermute_3) -> AIE to HLS10/1
  AIE/13(ToOutputPermute_4) -> AIE to HLS11/1
  AIE/14(ToOutputPermute_5) -> AIE to HLS13/1
  AIE/15(ToOutputPermute_6) -> AIE to HLS14/1
  AIE/16(ToOutputPermute_7) -> AIE to HLS12/1
  HLS to AIE/1 -> AIE/9(FromCyclicShift_0)
  HLS to AIE1/1 -> AIE/10(FromCyclicShift_1)
  HLS to AIE2/1 -> AIE/11(FromCyclicShift_2)
  HLS to AIE3/1 -> AIE/12(FromCyclicShift_3)
  HLS to AIE4/1 -> AIE/13(FromCyclicShift_4)
  HLS to AIE5/1 -> AIE/14(FromCyclicShift_5)
  HLS to AIE6/1 -> AIE/15(FromCyclicShift_6)
  HLS to AIE7/1 -> AIE/16(FromCyclicShift_7)
  AIE/5(ChannelizerOut_4) -> ChannelizerOut_4/1
  AIE/6(ChannelizerOut_5) -> ChannelizerOut_5/1
  AIE/7(ChannelizerOut_6) -> ChannelizerOut_6/1
  AIE/8(ChannelizerOut_7) -> ChannelizerOut_7/1
  AIE/4(ChannelizerOut_3) -> ChannelizerOut_3/1
  AIE/3(ChannelizerOut_2) -> ChannelizerOut_2/1
  AIE/2(ChannelizerOut_1) -> ChannelizerOut_1/1
  AIE/1(ChannelizerOut_0) -> ChannelizerOut_0/1
  AIE to HLS4/1 -> m16_ssr8_permute_fb_i_wrapper/4
  AIE to HLS7/1 -> m16_ssr8_permute_fb_i_wrapper/7
  m16_ssr8_permute_fb_i_wrapper/6 -> HLS to AIE13/1
  AIE to HLS1/1 -> m16_ssr8_permute_fb_i_wrapper/1
  AIE to HLS2/1 -> m16_ssr8_permute_fb_i_wrapper/2
  m16_ssr8_permute_fb_i_wrapper/7 -> HLS to AIE14/1
  AIE to HLS3/1 -> m16_ssr8_permute_fb_i_wrapper/3
  m16_ssr8_permute_fb_i_wrapper/8 -> HLS to AIE15/1
  m16_ssr8_permute_fb_i_wrapper/5 -> HLS to AIE12/1
  AIE to HLS6/1 -> m16_ssr8_permute_fb_i_wrapper/6
  m16_ssr8_permute_fb_i_wrapper/3 -> HLS to AIE10/1
  m16_ssr8_permute_fb_i_wrapper/1 -> HLS to AIE8/1
  m16_ssr8_permute_fb_i_wrapper/4 -> HLS to AIE11/1
  AIE to HLS5/1 -> m16_ssr8_permute_fb_i_wrapper/5
  m16_ssr8_permute_fb_i_wrapper/2 -> HLS to AIE9/1
  AIE to HLS/1 -> m16_ssr8_permute_fb_o_wrapper/1
  AIE to HLS8/1 -> m16_ssr8_permute_fb_o_wrapper/2
  AIE to HLS9/1 -> m16_ssr8_permute_fb_o_wrapper/3
  AIE to HLS10/1 -> m16_ssr8_permute_fb_o_wrapper/4
  AIE to HLS11/1 -> m16_ssr8_permute_fb_o_wrapper/5
  AIE to HLS13/1 -> m16_ssr8_permute_fb_o_wrapper/6
  AIE to HLS14/1 -> m16_ssr8_permute_fb_o_wrapper/7
  AIE to HLS12/1 -> m16_ssr8_permute_fb_o_wrapper/8
  m16_ssr8_permute_fb_o_wrapper/1 -> m16_ssr8_cyclic_shift_wrapper/1
  m16_ssr8_permute_fb_o_wrapper/2 -> m16_ssr8_cyclic_shift_wrapper/2
  m16_ssr8_permute_fb_o_wrapper/3 -> m16_ssr8_cyclic_shift_wrapper/3
  m16_ssr8_permute_fb_o_wrapper/4 -> m16_ssr8_cyclic_shift_wrapper/4
  m16_ssr8_permute_fb_o_wrapper/5 -> m16_ssr8_cyclic_shift_wrapper/5
  m16_ssr8_permute_fb_o_wrapper/6 -> m16_ssr8_cyclic_shift_wrapper/6
  m16_ssr8_permute_fb_o_wrapper/7 -> m16_ssr8_cyclic_shift_wrapper/7
  m16_ssr8_permute_fb_o_wrapper/8 -> m16_ssr8_cyclic_shift_wrapper/8
  ChannelizerIn_0/1 -> AIE to HLS1/1
  ChannelizerIn_1/1 -> AIE to HLS2/1
  ChannelizerIn_2/1 -> AIE to HLS3/1
  ChannelizerIn_3/1 -> AIE to HLS4/1
  ChannelizerIn_4/1 -> AIE to HLS5/1
  ChannelizerIn_5/1 -> AIE to HLS6/1
  ChannelizerIn_6/1 -> AIE to HLS7/1
  HLS to AIE8/1 -> AIE/1(FromInputPermute_0)
  HLS to AIE9/1 -> AIE/2(FromInputPermute_1)
  HLS to AIE10/1 -> AIE/3(FromInputPermute_2)
  HLS to AIE11/1 -> AIE/4(FromInputPermute_3)
  HLS to AIE12/1 -> AIE/5(FromInputPermute_4)
  HLS to AIE13/1 -> AIE/6(FromInputPermute_5)
  HLS to AIE14/1 -> AIE/7(FromInputPermute_6)
  HLS to AIE15/1 -> AIE/8(FromInputPermute_7)

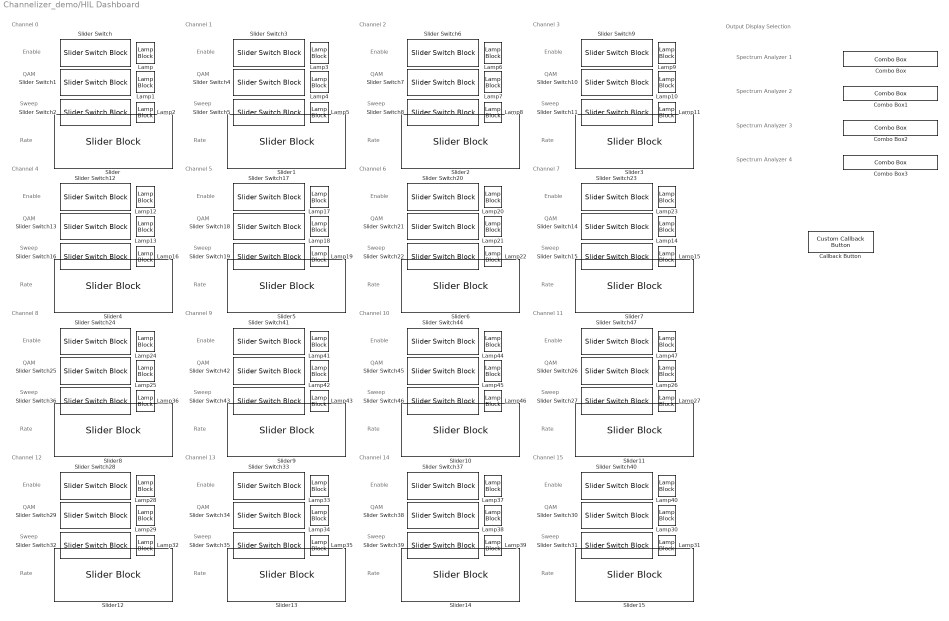
== system Channelizer_demo/HIL Dashboard ==
  note: Output Display Selection
  note: Spectrum Analyzer 1
  note: Enable
  note: Channel 0
  note: QAM
  note: Sweep
  note: Rate
  note: Channel 1
  note: Rate
  note: QAM
  note: Sweep
  note: Enable
  note: Channel 2
  note: Channel 3
  note: Rate
  note: Enable
  note: QAM
  note: Sweep
  note: QAM
  note: Sweep
  note: Rate
  note: Enable
  note: QAM
  note: Enable
  note: Rate
  note: Sweep
  note: Rate
  note: Sweep
  note: Sweep
  note: Channel 5
  note: Channel 6
  note: Rate
  note: Enable
  note: Channel 7
  note: QAM
  note: Sweep
  note: Channel 4
  note: Enable
  note: Enable
  note: QAM
  note: Rate
  note: QAM
  note: Rate
  note: Rate
  note: Sweep
  note: Enable
  note: Rate
  note: Enable
  note: QAM
  note: QAM
  note: Sweep
  note: Channel 11
  note: Sweep
  note: QAM
  note: Rate
  note: Enable
  note: Channel 10
  note: Channel 12
  note: Channel 15
  note: Enable
  note: Enable
  note: Channel 8
  note: QAM
  note: Rate
  note: Sweep
  note: Sweep
  note: QAM
  note: Rate
  note: Channel 14
  note: Enable
  note: QAM
  note: Channel 9
  note: Sweep
  note: QAM
  note: Enable
  note: Sweep
  note: Rate
  note: Sweep
  note: Rate
  note: Channel 13
  note: Enable
  note: QAM
  note: Spectrum Analyzer 2
  note: Spectrum Analyzer 3
  note: Spectrum Analyzer 4
  Callback Button : CustomCallbackButton  Configuration="{\"components\":[{\"name\":\"BackgroundImageComponent\",\"settings\":{\"image\":{\"size\":[0,0],\"src\":\"default\",\"srcOrientation\":\"Right\"},\"position\":[0,0,1,1]}},{\"name\":\"ButtonStateComponent\",\"settings\":{\"buttonType\":\"momentary\",\"clickFcn\":\"channelizer_demo_init;\",\"onValue\":1,\"position\":[0,0,1,1],\"pressDelay\":\"500\",\"pressFcn\":\"\",\"repeatInterval\":\"0\",\"states\":[{\"horizontalAlignment\":\"center\",\"image\":{\"position\":[0,0,1,1],\"size\":[1,1],\"src\":\"default\",\"srcOrientation\":\"Right\"},\"label\":{\"color\":[1,1,1],\"icon\":{\"size\":[0,0],\"src\":\"default\",\"srcOrientation\":\"Right\"},\"iconPlacement\":\"left\",\"opacity\":1,\"show\":true,\"text\":{\"content\":\"RESET\",\"font\":\"Helvetica\",\"fontSize\":12}},\"labelOffset\":[0,0],\"verticalAlignment\":\"middle\"},{\"horizontalAlignment\":\"center\",\"image\":{\"position\":[0,0,1,1],\"size\":[1,1],\"src\":\"default\",\"srcOrientation\":\"Right\"},\"label\":{\"color\":[1,1,1],\"icon\":{\"size\":[0,0],\"src\":\"default\",\"srcOrientation\":\"Right\"},\"iconPlacement\":\"left\",\"opacity\":1,\"show\":true,\"text\":{\"content\":\"RESET\",\"font\":\"Helvetica\",\"fontSize\":12}},\"labelOffset\":[0,0],\"verticalAlignment\":\"middle\"},{\"horizontalAlignment\":\"center\",\"image\":{\"position\":[0,0,1,1],\"size\":[1,1],\"src\":\"default\",\"srcOrientation\":\"Right\"},\"label\":{\"color\":[1,1,1],\"icon\":{\"size\":[0,0],\"src\":\"default\",\"srcOrientation\":\"Right\"},\"iconPlacement\":\"left\",\"opacity\":1,\"show\":true,\"text\":{\"content\":\"RESET\",\"font\":\"Helvetica\",\"fontSize\":12}},\"labelOffset\":[0,0],\"verticalAlignment\":\"middle\"},{\"horizontalAlignment\":\"center\",\"image\":{\"position\":[0,0,1,1],\"size\":[1,1],\"src\":\"default\",\"srcOrientation\":\"Right\"},\"label\":{\"color\":[1,1,1],\"icon\":{\"size\":[0,0],\"src\":\"default\",\"srcOrientation\":\"Right\"},\"iconPlacement\":\"left\",\"opacity\":1,\"show\":true,\"text\":{\"content\":\"RESET\",\"font\":\"Helvetica\",\"fontSize\":12}},\"labelOffset\":[0,0],\"verticalAlignment\":\"middle\"}]}},{\"name\":\"ForegroundImageComponent\",\"settings\":{\"image\":{\"size\":[0,0],\"src\":\"default\",\"srcOrientation\":\"Right\"},\"isForeground\":1,\"position\":[0,0,1,1]}}],\"settings\":{\"BindingType\":\"standalone\",\"backgroundColor\":[244,244,244,1],\"backgroundOffset\":0.2,\"backgroundOpacity\":1,\"fixedAspectRatio\":\"on\",\"foregroundColor\":[0.01176470588,0.01176470588,0.01176470588,1],\"migratedFromLegacy\":true,\"useBackgroundColor\":true,\"variant\":\"callback\",\"version\":\"R2023a\"},\"type\":\"Button\"}"  CustomBackgroundColor="{\"color\":[0,0.447059,0.741176],\"show\":true}"
  Combo Box : ComboBox  LabelPosition=Hide  SelectedLabel=Channel 1
      settings: Values={{'Channel 0', 'Channel 1', 'Channel 2', 'Channel 3', 'Channel 4', 'Channel 5', 'Channel 6', 'Channel 7', 'Channel 8', 'Channel 9', 'Channel 10', 'Channel 11', 'Channel 12', 'Channel 13', 'Channel 14', 'Channel 15'}, [0 1 2 3 4 5 6 7 8 9 10 11 12 13 14 15]}
  Combo Box1 : ComboBox  LabelPosition=Hide  SelectedLabel=Channel 2
      settings: Values={{'Channel 0', 'Channel 1', 'Channel 2', 'Channel 3', 'Channel 4', 'Channel 5', 'Channel 6', 'Channel 7', 'Channel 8', 'Channel 9', 'Channel 10', 'Channel 11', 'Channel 12', 'Channel 13', 'Channel 14', 'Channel 15'}, [0 1 2 3 4 5 6 7 8 9 10 11 12 13 14 15]}
  Combo Box2 : ComboBox  LabelPosition=Hide  SelectedLabel=Channel 5
      settings: Values={{'Channel 0', 'Channel 1', 'Channel 2', 'Channel 3', 'Channel 4', 'Channel 5', 'Channel 6', 'Channel 7', 'Channel 8', 'Channel 9', 'Channel 10', 'Channel 11', 'Channel 12', 'Channel 13', 'Channel 14', 'Channel 15'}, [0 1 2 3 4 5 6 7 8 9 10 11 12 13 14 15]}
  Combo Box3 : ComboBox  LabelPosition=Hide  SelectedLabel=Channel 6
      settings: Values={{'Channel 0', 'Channel 1', 'Channel 2', 'Channel 3', 'Channel 4', 'Channel 5', 'Channel 6', 'Channel 7', 'Channel 8', 'Channel 9', 'Channel 10', 'Channel 11', 'Channel 12', 'Channel 13', 'Channel 14', 'Channel 15'}, [0 1 2 3 4 5 6 7 8 9 10 11 12 13 14 15]}
  Lamp{,1..47} (48 alike) : LampBlock  LabelPosition=Hide
  Slider{,1..3} (4 alike) : SliderBlock  LabelPosition=Hide  ScaleMin=-0.1  ScaleMax=0.1
  Slider Switch{,1..47} (48 alike) : SliderSwitchBlock  LabelPosition=Hide
      settings: Values={{'Off', 'On'}, [0 1]}
  Slider{8..11} (4 alike) : SliderBlock  LabelPosition=Hide  ScaleMin=-1  ScaleMax=1
  Slider{12..15} (4 alike) : SliderBlock  LabelPosition=Hide  ScaleMin=-5  ScaleMax=5
  Slider{4..7} (4 alike) : SliderBlock  LabelPosition=Hide  ScaleMin=-0.5  ScaleMax=0.5

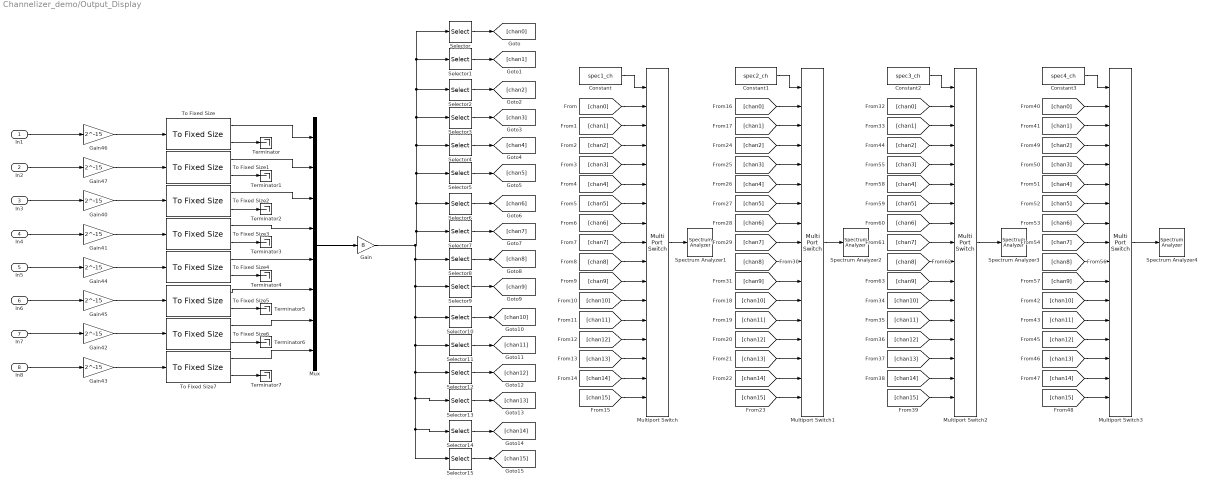
== system Channelizer_demo/Output_Display ==
  In1 : Inport
  In2 : Inport  Port=2
  In3 : Inport  Port=3
  In4 : Inport  Port=4
  In5 : Inport  Port=5
  In6 : Inport  Port=6
  In7 : Inport  Port=7
  In8 : Inport  Port=8
  Constant : Constant  Value=spec1_ch  SampleTime=-1
  Constant1 : Constant  Value=spec2_ch  SampleTime=-1
  Constant2 : Constant  Value=spec3_ch  SampleTime=-1
  Constant3 : Constant  Value=spec4_ch  SampleTime=-1
  Gain : Gain  Gain=8
  Gain{40..47} (8 alike) : Gain  Gain=2^-15  OutDataTypeStr=double
  Multiport Switch{,1..3} (4 alike) : MultiPortSwitch  DataPortOrder=Zero-based contiguous  Inputs=16  zeroidx=on  SaturateOnIntegerOverflow=off  InputSameDT=off
  Mux : Mux  Inputs=8
  Selector : Selector  InputPortWidth=32  IndexOptions=Index vector (dialog)  Indices=[1 5]  OutputSizes=1
  Selector1 : Selector  InputPortWidth=32  IndexOptions=Index vector (dialog)  Indices=[2 6]  OutputSizes=1
  Selector10 : Selector  InputPortWidth=32  IndexOptions=Index vector (dialog)  Indices=[19 23]  OutputSizes=1
  Selector11 : Selector  InputPortWidth=32  IndexOptions=Index vector (dialog)  Indices=[20 24]  OutputSizes=1
  Selector12 : Selector  InputPortWidth=32  IndexOptions=Index vector (dialog)  Indices=[25 29]  OutputSizes=1
  Selector13 : Selector  InputPortWidth=32  IndexOptions=Index vector (dialog)  Indices=[26 30]  OutputSizes=1
  Selector14 : Selector  InputPortWidth=32  IndexOptions=Index vector (dialog)  Indices=[27 31]  OutputSizes=1
  Selector15 : Selector  InputPortWidth=32  IndexOptions=Index vector (dialog)  Indices=[28 32]  OutputSizes=1
  Selector2 : Selector  InputPortWidth=32  IndexOptions=Index vector (dialog)  Indices=[3 7]  OutputSizes=1
  Selector3 : Selector  InputPortWidth=32  IndexOptions=Index vector (dialog)  Indices=[4 8]  OutputSizes=1
  Selector4 : Selector  InputPortWidth=32  IndexOptions=Index vector (dialog)  Indices=[9 13]  OutputSizes=1
  Selector5 : Selector  InputPortWidth=32  IndexOptions=Index vector (dialog)  Indices=[10 14]  OutputSizes=1
  Selector6 : Selector  InputPortWidth=32  IndexOptions=Index vector (dialog)  Indices=[11 15]  OutputSizes=1
  Selector7 : Selector  InputPortWidth=32  IndexOptions=Index vector (dialog)  Indices=[12 16]  OutputSizes=1
  Selector8 : Selector  InputPortWidth=32  IndexOptions=Index vector (dialog)  Indices=[17 21]  OutputSizes=1
  Selector9 : Selector  InputPortWidth=32  IndexOptions=Index vector (dialog)  Indices=[18 22]  OutputSizes=1
  Spectrum Analyzer1 : SpectrumAnalyzer  WindowPosition=[2001.000000,1029.000000,557.000000,293.000000,]  Visible=on  ScopeFrameLocation=window  AxesScaling=Manual  Span=625000000  StartFrequency=-312500000  StopFrequency=312500000  AveragingMethod=Exponential  YLimits=[-52.56925268,41.63226586]
  Spectrum Analyzer2 : SpectrumAnalyzer  WindowPosition=[2002.000000,696.000000,557.000000,293.000000,]  Visible=on  ScopeFrameLocation=window  AxesScaling=Manual  Span=625000000  StartFrequency=-312500000  StopFrequency=312500000  AveragingMethod=Exponential  YLimits=[-52.56925268,41.63226586]
  Spectrum Analyzer3 : SpectrumAnalyzer  WindowPosition=[2002.000000,361.000000,557.000000,293.000000,]  Visible=on  ScopeFrameLocation=window  AxesScaling=Manual  Span=625000000  StartFrequency=-312500000  StopFrequency=312500000  AveragingMethod=Exponential  YLimits=[-52.56925268,41.63226586]  SelectedToolstripTab=spectrumAnalyzerToolstrip.estimationTab
  Spectrum Analyzer4 : SpectrumAnalyzer  WindowPosition=[2002.000000,33.000000,557.000000,293.000000,]  Visible=on  ScopeFrameLocation=window  AxesScaling=Manual  Span=625000000  StartFrequency=-312500000  StopFrequency=312500000  AveragingMethod=Exponential  YLimits=[-52.56925268,41.63226586]  SelectedToolstripTab=spectrumAnalyzerToolstrip.estimationTab
  Terminator{,1..7} (8 alike) : Terminator
  To Fixed Size{,1..7} (8 alike) : aieUtilities/To Fixed Size  Mode=Produce a valid output signal  OutputSize=Inherit: Same as input  CopyMethod=Buffer samples to form output  HasStatusOutput=on
  wires:
  In8/1 -> Gain43/1
  In5/1 -> Gain44/1
  In3/1 -> Gain40/1
  In6/1 -> Gain45/1
  In4/1 -> Gain41/1
  In2/1 -> Gain47/1
  Gain42/1 -> To Fixed Size6/1
  Gain41/1 -> To Fixed Size3/1
  Gain44/1 -> To Fixed Size4/1
  Gain40/1 -> To Fixed Size2/1
  Gain46/1 -> To Fixed Size/1
  Gain45/1 -> To Fixed Size5/1
  Gain47/1 -> To Fixed Size1/1
  In1/1 -> Gain46/1
  Gain43/1 -> To Fixed Size7/1
  In7/1 -> Gain42/1
  To Fixed Size/2 -> Terminator/1
  To Fixed Size1/2 -> Terminator1/1
  To Fixed Size2/2 -> Terminator2/1
  To Fixed Size3/2 -> Terminator3/1
  To Fixed Size4/2 -> Terminator4/1
  To Fixed Size5/2 -> Terminator5/1
  To Fixed Size6/2 -> Terminator6/1
  To Fixed Size7/2 -> Terminator7/1
  To Fixed Size7/1 -> Mux/8
  To Fixed Size6/1 -> Mux/7
  To Fixed Size5/1 -> Mux/6
  To Fixed Size4/1 -> Mux/5
  To Fixed Size3/1 -> Mux/4
  To Fixed Size2/1 -> Mux/3
  To Fixed Size1/1 -> Mux/2
  To Fixed Size/1 -> Mux/1
  Mux/1 -> Gain/1
  Selector/1 -> [chan0]
  Selector1/1 -> [chan1]
  Selector3/1 -> [chan3]
  Selector2/1 -> [chan2]
  Selector7/1 -> [chan7]
  Selector6/1 -> [chan6]
  Selector5/1 -> [chan5]
  Selector4/1 -> [chan4]
  Selector15/1 -> [chan15]
  Selector14/1 -> [chan14]
  Selector13/1 -> [chan13]
  Selector12/1 -> [chan12]
  Selector11/1 -> [chan11]
  Selector10/1 -> [chan10]
  Selector9/1 -> [chan9]
  Selector8/1 -> [chan8]
  Gain/1 -> Selector13/1, Selector14/1, Selector15/1, Selector12/1, Selector11/1, Selector10/1, Selector9/1, Selector8/1, Selector6/1, Selector4/1, Selector3/1, Selector2/1, Selector1/1, Selector/1, Selector5/1, Selector7/1
  [chan15] -> Multiport Switch/17
  [chan14] -> Multiport Switch/16
  [chan13] -> Multiport Switch/15
  [chan12] -> Multiport Switch/14
  [chan11] -> Multiport Switch/13
  [chan4] -> Multiport Switch/6
  [chan5] -> Multiport Switch/7
  [chan6] -> Multiport Switch/8
  [chan7] -> Multiport Switch/9
  [chan10] -> Multiport Switch/12
  [chan9] -> Multiport Switch/11
  [chan8] -> Multiport Switch/10
  [chan3] -> Multiport Switch/5
  [chan2] -> Multiport Switch/4
  [chan1] -> Multiport Switch/3
  [chan0] -> Multiport Switch/2
  Multiport Switch/1 -> Spectrum Analyzer1/1
  Constant/1 -> Multiport Switch/1
  [chan1] -> Multiport Switch1/3
  [chan15] -> Multiport Switch1/17
  [chan5] -> Multiport Switch1/7
  [chan14] -> Multiport Switch1/16
  [chan3] -> Multiport Switch1/5
  [chan2] -> Multiport Switch1/4
  [chan6] -> Multiport Switch1/8
  [chan7] -> Multiport Switch1/9
  [chan12] -> Multiport Switch1/14
  Multiport Switch1/1 -> Spectrum Analyzer2/1
  [chan0] -> Multiport Switch1/2
  [chan4] -> Multiport Switch1/6
  [chan9] -> Multiport Switch1/11
  [chan10] -> Multiport Switch1/12
  [chan8] -> Multiport Switch1/10
  [chan11] -> Multiport Switch1/13
  Constant1/1 -> Multiport Switch1/1
  [chan13] -> Multiport Switch1/15
  [chan1] -> Multiport Switch3/3
  [chan8] -> Multiport Switch3/10
  [chan8] -> Multiport Switch2/10
  [chan4] -> Multiport Switch3/6
  Multiport Switch3/1 -> Spectrum Analyzer4/1
  [chan0] -> Multiport Switch2/2
  [chan14] -> Multiport Switch2/16
  [chan3] -> Multiport Switch2/5
  [chan9] -> Multiport Switch3/11
  [chan0] -> Multiport Switch3/2
  [chan15] -> Multiport Switch2/17
  [chan10] -> Multiport Switch3/12
  [chan9] -> Multiport Switch2/11
  [chan6] -> Multiport Switch2/8
  Constant3/1 -> Multiport Switch3/1
  [chan1] -> Multiport Switch2/3
  [chan7] -> Multiport Switch2/9
  [chan14] -> Multiport Switch3/16
  [chan4] -> Multiport Switch2/6
  [chan7] -> Multiport Switch3/9
  [chan15] -> Multiport Switch3/17
  [chan10] -> Multiport Switch2/12
  [chan3] -> Multiport Switch3/5
  [chan13] -> Multiport Switch3/15
  Constant2/1 -> Multiport Switch2/1
  [chan5] -> Multiport Switch3/7
  [chan5] -> Multiport Switch2/7
  Multiport Switch2/1 -> Spectrum Analyzer3/1
  [chan12] -> Multiport Switch2/14
  [chan2] -> Multiport Switch2/4
  [chan2] -> Multiport Switch3/4
  [chan6] -> Multiport Switch3/8
  [chan11] -> Multiport Switch2/13
  [chan13] -> Multiport Switch2/15
  [chan11] -> Multiport Switch3/13
  [chan12] -> Multiport Switch3/14
